simulink model "Cell_balancing"  (R2021a)
settings: Solver=VariableStepAuto  StartTime=0.0  StopTime=10.0  RelTol=1e-3
undefined symbols (not defined in the file or in its folder): Ion, Lithium
libraries: spsMosfetLib x6, spsBatteryLib x3, eePwmGenerator x2, spsSeriesRLCBranchLib x1, spsVoltageMeasurementLib x1, spspowerguiLib x1
settings Model: Creator=sampa  LastModifiedBy=sampa

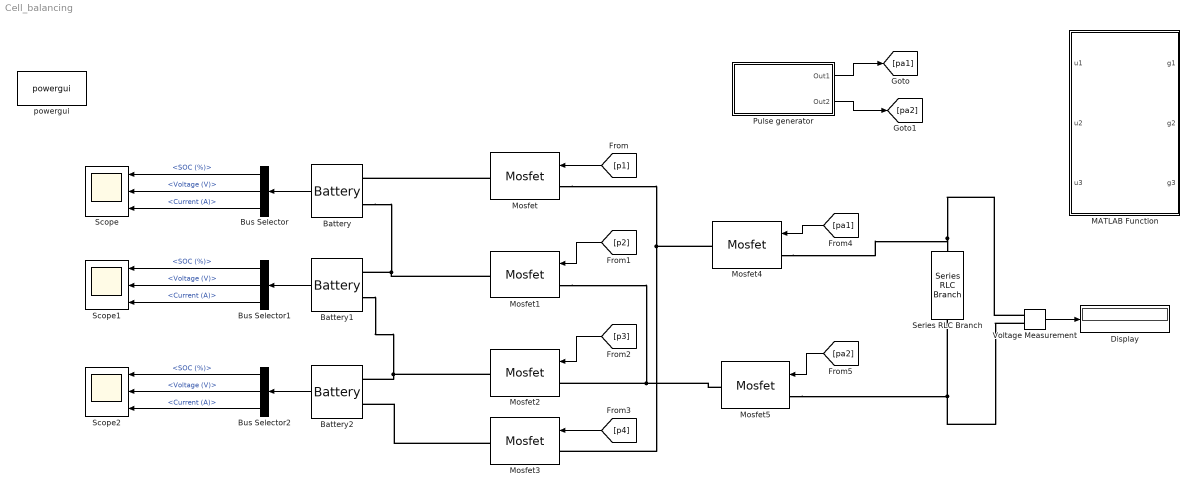
== system Cell_balancing ==
  Battery : spsBatteryLib/Battery  BatType=Lithium-Ion  ShowTempParam=off  ThermalPreset=no  ShowAgeParam=off  NomV=3.4  NomQ=4.2  SOC=50  Batt_Tr=30  PresetModel=on  MaxQ=4.2  MinV=2.55  FullV=3.9576  Dis_rate=1.8261  R=0.0080952  Normal_OP=3.7983  expZone="[3.6733     0.20635]"  current=[6.5 13 32.5]  Units=Time  Tci=20  NomT=20  T2=-30  MaxQ2=4.8  FullV2=7.1  Normal_OP2=5.655  expZone2="[6.58           1]"  Rca=0.6  ti=2000  Dp=0  Neq0=0  Tsim=1e6  Ta1=25  Qeol=5.4*0.9  Reol=0.013333*1.2  Char_age=[2.3478, 3]  Dis_age=[2.3478, 10]  N1=1500  N2=10500  N3=1000  N4=1400  Ta2=45  N5=950
  Battery1 : spsBatteryLib/Battery  BatType=Lithium-Ion  ShowTempParam=off  ThermalPreset=no  ShowAgeParam=off  NomV=3.6  NomQ=4.2  SOC=30  Batt_Tr=30  PresetModel=on  MaxQ=4.2  MinV=2.7  FullV=4.1904  Dis_rate=1.8261  R=0.0085714  Normal_OP=3.7983  expZone="[3.8894     0.20635]"  current=[6.5 13 32.5]  Units=Time  Tci=20  NomT=20  T2=-30  MaxQ2=4.8  FullV2=7.1  Normal_OP2=5.655  expZone2="[6.58           1]"  Rca=0.6  ti=2000  Dp=0  Neq0=0  Tsim=1e6  Ta1=25  Qeol=5.4*0.9  Reol=0.013333*1.2  Char_age=[2.3478, 3]  Dis_age=[2.3478, 10]  N1=1500  N2=10500  N3=1000  N4=1400  Ta2=45  N5=950
  Battery2 : spsBatteryLib/Battery  BatType=Lithium-Ion  ShowTempParam=off  ThermalPreset=no  ShowAgeParam=off  NomV=3.6  NomQ=4.2  SOC=75  Batt_Tr=30  PresetModel=on  MaxQ=4.2  MinV=2.7  FullV=4.1904  Dis_rate=1.8261  R=0.0085714  Normal_OP=3.7983  expZone="[3.8894     0.20635]"  current=[6.5 13 32.5]  Units=Time  Tci=20  NomT=20  T2=-30  MaxQ2=4.8  FullV2=7.1  Normal_OP2=5.655  expZone2="[6.58           1]"  Rca=0.6  ti=2000  Dp=0  Neq0=0  Tsim=1e6  Ta1=25  Qeol=5.4*0.9  Reol=0.013333*1.2  Char_age=[2.3478, 3]  Dis_age=[2.3478, 10]  N1=1500  N2=10500  N3=1000  N4=1400  Ta2=45  N5=950
  Bus Selector : BusSelector  OutputSignals=SOC (%),Voltage (V),Current (A)
  Bus Selector1 : BusSelector  OutputSignals=SOC (%),Voltage (V),Current (A)
  Bus Selector2 : BusSelector  OutputSignals=SOC (%),Voltage (V),Current (A)
  Display : Display
  MATLAB Function : MATLAB Function  TreatAsAtomicUnit=on
  Mosfet{,1..5} (6 alike) : spsMosfetLib/Mosfet  Ron=0.1  Lon=0  Rd=0.01  Vfd=0  IC=0  Rs=1e5  Cs=inf  Measurements=off
  Pulse generator : Subsystem
  Scope : Scope  NumInputPorts=3
  Scope1 : Scope  NumInputPorts=3
  Scope2 : Scope  NumInputPorts=3
  Series RLC Branch : spsSeriesRLCBranchLib/Series RLC Branch  LConnTagsString=__new0  RConnTagsString=__new0  BranchType=R  Resistance=1  Inductance=1e-3  SetiL0=off  InitialCurrent=0  Capacitance=1e-6  Setx0=off  InitialVoltage=0  Measurements=None
  Voltage Measurement : spsVoltageMeasurementLib/Voltage Measurement  PhasorSimulation=off  OutputType=Complex  PSBequivalent=0
  powergui : spspowerguiLib/powergui  Priority=1  SimulationMode=Continuous  SampleTime=50e-6  frequency=60  Iterations=50  frequencyindice=0  Pbase=100e6  ErrMax=1e-4  UnitsV=kV  UnitsW=MW  buscounter=0  FunctionMessages=off  echomessages=off  EnableUseOfTLC=off  CurrentSourceSwitches=off  DisableSnubberDevices=off  DisableRonSwitches=off  DisableVfSwitches=off  DisplayEquations=off  AutomaticDiscreteSolvers=off  SolverType=Tustin/Backward Euler (TBE)  Interpol=off  ExternalGateDelay=off  methode=off  Ts=100  x0status=blocks  SPID=on  SwTol=0  HookPort=off  NonlinearTolerance=1e-4  nMaxIteration=100  ContinueOnMaxIteration=off  RestoreLinks=warning  ResistiveCurrentMeasurement=off  Frange=[0:2:500]  Ylog=off  Xlog=on  ShowGrid=off  save=off  variable=ZData  structure=0  ZoomFFT=off  StartTime=0.0  cycles=1  DisplayStyle=1  fundamental=60  FreqAxis=off  MaxFrequency=1000  frequencyindicesteady=1  RmsSteady=1  display=off
  wires:
  Battery/1 -> Bus Selector/1
  Bus Selector/1 -> Scope/1  "<SOC (%)>"
  [p2] -> Mosfet1/1
  [p1] -> Mosfet/1
  [p3] -> Mosfet2/1
  Voltage Measurement/1 -> Display/1
  [pa2] -> Mosfet5/1
  [p4] -> Mosfet3/1
  [pa1] -> Mosfet4/1
  Bus Selector/2 -> Scope/2  "<Voltage (V)>"
  Bus Selector/3 -> Scope/3  "<Current (A)>"
  Bus Selector1/2 -> Scope1/2  "<Voltage (V)>"
  Bus Selector1/3 -> Scope1/3  "<Current (A)>"
  Battery1/1 -> Bus Selector1/1
  Bus Selector1/1 -> Scope1/1  "<SOC (%)>"
  Bus Selector2/2 -> Scope2/2  "<Voltage (V)>"
  Bus Selector2/3 -> Scope2/3  "<Current (A)>"
  Battery2/1 -> Bus Selector2/1
  Bus Selector2/1 -> Scope2/1  "<SOC (%)>"
  Pulse generator/1(Out1) -> [pa1]
  Pulse generator/2(Out2) -> [pa2]
  connections:
  Battery/LConn2 -- Battery1/LConn1 -- Mosfet1/RConn1
  Battery1/LConn2 -- Battery2/LConn1 -- Mosfet2/RConn1
  Mosfet/RConn1 -- Battery/LConn1
  Voltage Measurement/LConn1 -- Mosfet4/LConn1 -- Series RLC Branch/RConn1
  Mosfet3/RConn1 -- Battery2/LConn2
  Voltage Measurement/LConn2 -- Mosfet5/LConn1 -- Series RLC Branch/LConn1
  Mosfet1/LConn1 -- Mosfet2/LConn1 -- Mosfet5/RConn1
  Mosfet/LConn1 -- Mosfet4/RConn1 -- Mosfet3/LConn1

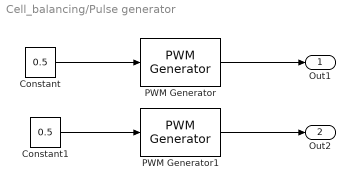
== system Cell_balancing/Pulse generator ==
  Constant : Constant  Value=0.5
  Constant1 : Constant  Value=0.5
  PWM Generator : eePwmGenerator/PWM Generator  CarrCount=Up  Tper=0.001  Ts=5e-5
  PWM Generator1 : eePwmGenerator/PWM Generator  CarrCount=Up  Tper=0.001  Ts=5e-5
  Out1 : Outport
  Out2 : Outport  Port=2
  wires:
  PWM Generator/1 -> Out1/1
  PWM Generator1/1 -> Out2/1
  Constant/1 -> PWM Generator/1
  Constant1/1 -> PWM Generator1/1

== matlab function Cell_balancing/MATLAB Function ==
  data: u1 input; g1 output; u2 input; u3 input; g2 output; g3 output
 function [g1,g2,g3] = fcn(u1,u2,u3)

u1 = u1*1000;
u2 = u2*1000;
u3 = u3*1000;

u1 = int32(u1);
u2 = int32(u2);
u3 = int32(u3);

if u1>u2||u1>u3
    g1 = 1;
else g1 = 0;
end
 if u2>u1||u2>u3
     g2 = 1;
 else g2 = 0;
 end
     if u3>u1||u3>u2
         g3 = 1;
     else g3 = 0;
     end
